simulink model "三相配电系统仿真模型"  (R2024b)
settings: Solver=VariableStepAuto  StartTime=0.0  StopTime=0.5  RelTol=1e-3
libraries: spsCurrentMeasurementLib x18, spsVoltageMeasurementLib x18, spsGroundLib x6, spsThreePhaseSeriesRLCBranchLib x2, spsThreePhaseTransformerThreeWindingsLib x2, spsThreePhaseSeriesRLCLoadLib x1, spsThreePhaseSourceLib x1, sps_lib x1
settings Model: Creator=Land  LastModifiedBy=MihoLocal
settings SFSimCC: UsePrecompiledLibraries=Avoid  SimTargetLang=C++  GPUAcceleration=on  SimDLTargetLibrary=cudnn

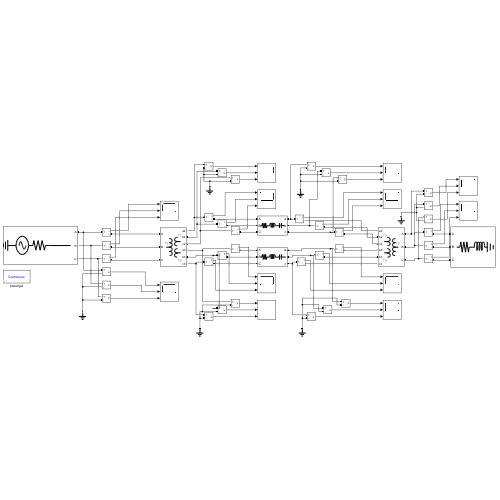
[thumbnail: Simulink's stored preview of the top-level diagram]
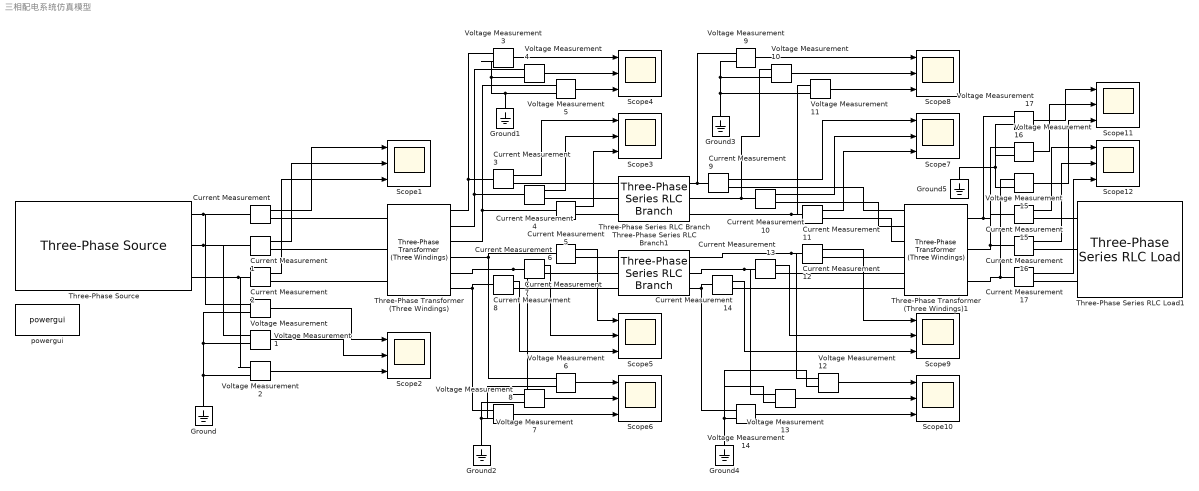
== system 三相配电系统仿真模型 ==
  Current Measurement{,1..17} (18 alike) : spsCurrentMeasurementLib/Current Measurement  PhasorSimulation=off  OutputType=Complex  PSBequivalent=0
  Ground{,1..5} (6 alike) : spsGroundLib/Ground  LConnTagsString=a
  Scope{1..12} (12 alike) : Scope  NumInputPorts=3
  Three-Phase Series RLC Branch : spsThreePhaseSeriesRLCBranchLib/Three-Phase Series RLC Branch  LConnTagsString=A|B|C  RConnTagsString=A|B|C  BranchType=RLC  Resistance=5  Inductance=1e-3  Capacitance=0  Measurements=None
  Three-Phase Series RLC Branch1 : spsThreePhaseSeriesRLCBranchLib/Three-Phase Series RLC Branch  LConnTagsString=A|B|C  RConnTagsString=A|B|C  BranchType=RLC  Resistance=5  Inductance=1e-3  Capacitance=1e-3  Measurements=None
  Three-Phase Series RLC Load1 : spsThreePhaseSeriesRLCLoadLib/Three-Phase Series RLC Load  LConnTagsString=A|B|C  Configuration=Y (grounded)  NominalVoltage=30  Vabc=[1e3 1e3 1e3]  Vabcp=[1e3 1e3 1e3]  NominalFrequency=50  UnbalancedPower=off  ActivePower=10e3  InductivePower=1  CapacitivePower=0  Pabc=[10e3 9e3 11e3]  QLabc=[100 90 110]  QCabc=[100 90 110]  Pabcp=[10e3 9e3 11e3]  QLabcp=[100 90 110]  QCabcp=[100 90 110]  Measurements=None  LoadType=constant Z
  Three-Phase Transformer (Three Windings) : spsThreePhaseTransformerThreeWindingsLib/Three-Phase Transformer (Three Windings)  Winding1Connection=Yg  Winding2Connection=Yg  Winding3Connection=Yg  CoreType=Three single-phase transformers  SetSaturation=off  Hysteresis=off  DataFile='hysteresis'  SetInitialFlux=off  Measurements=None  UNITS=pu  NominalPower=[ 24 , 50 ]  Winding1=[ 12 , 0.002 , 0.08 ]  Winding2=[ 12 , 0.002 , 0.08 ]  Winding3=[ 12 , 0.002 , 0.08 ]  Rm=500  Lm=500  L0=0.5  Saturation=[ 0,0 ; 0.0024,1.2 ; 1.0,1.52 ]  InitialFluxes=[0.8 -0.8 0.7]  BreakLoop=off  DiscreteSolver=Trapezoidal iterative  DataType=off  TransfoNumber=1
      settings: LibrarySourceBlock=|
      | sps_lib/Power Grid Elements/Three-Phase
      | Transformer
      | (Three Windings)
  Three-Phase Transformer (Three Windings)1 : spsThreePhaseTransformerThreeWindingsLib/Three-Phase Transformer (Three Windings)  Winding1Connection=Yg  Winding2Connection=Yg  Winding3Connection=Yg  CoreType=Three single-phase transformers  SetSaturation=off  Hysteresis=off  DataFile='hysteresis'  SetInitialFlux=off  Measurements=None  UNITS=pu  NominalPower=[ 24 , 50 ]  Winding1=[ 12 , 0.002 , 0.08 ]  Winding2=[ 12 , 0.002 , 0.08 ]  Winding3=[ 12 , 0.002 , 0.08 ]  Rm=500  Lm=500  L0=0.5  Saturation=[ 0,0 ; 0.0024,1.2 ; 1.0,1.52 ]  InitialFluxes=[0.8 -0.8 0.7]  BreakLoop=off  DiscreteSolver=Trapezoidal iterative  DataType=off  TransfoNumber=1
      settings: LibrarySourceBlock=|
      | sps_lib/Power Grid Elements/Three-Phase
      | Transformer
      | (Three Windings)
  Three-Phase Source : spsThreePhaseSourceLib/Three-Phase Source  InternalConnection=Yg  VoltagePhases=off  Voltage=12  PhaseAngle=0  Voltage_phases=[25e3 25e3 25e3]/sqrt(3)  PhaseAngles_phases=[0 -120 +120]  Frequency=50  NonIdealSource=on  SpecifyImpedance=off  Resistance=1  Inductance=0  ShortCircuitLevel=100e6  BaseVoltage=0  XRratio=7  BusType=swing  Pref=10e3  Qref=0  Prefabc=[10e3, 10e3, 10e3]  Qrefabc=[0, 0, 0]  Qmin=-inf  Qmax=inf
  Voltage Measurement{,1..17} (18 alike) : spsVoltageMeasurementLib/Voltage Measurement  PhasorSimulation=off  OutputType=Complex  PSBequivalent=0
  powergui : sps_lib/powergui  Priority=1  SimulationMode=Continuous  SampleTime=50e-6  frequency=60  Iterations=50  frequencyindice=50  Pbase=100e6  ErrMax=1e-4  UnitsV=kV  UnitsW=MW  buscounter=0  FunctionMessages=off  echomessages=off  EnableUseOfTLC=off  CurrentSourceSwitches=off  DisableSnubberDevices=off  DisableRonSwitches=off  DisableVfSwitches=off  DisplayEquations=off  AutomaticDiscreteSolvers=off  SolverType=Tustin/Backward Euler (TBE)  Interpol=off  ExternalGateDelay=off  methode=off  Ts=100  x0status=blocks  SPID=on  SwTol=0  HookPort=off  NonlinearTolerance=1e-4  nMaxIteration=100  ContinueOnMaxIteration=off  RestoreLinks=warning  ResistiveCurrentMeasurement=off  Frange=[0:2:500]  Ylog=off  Xlog=on  ShowGrid=off  save=off  variable=ZData  structure=0  ZoomFFT=off  StartTime=0.0  cycles=1  DisplayStyle=1  fundamental=60  FreqAxis=off  MaxFrequency=1000  frequencyindicesteady=1  RmsSteady=1  display=off
  wires:
  Current Measurement/1 -> Scope1/1
  Current Measurement1/1 -> Scope1/2
  Current Measurement2/1 -> Scope1/3
  Voltage Measurement/1 -> Scope2/1
  Voltage Measurement1/1 -> Scope2/2
  Voltage Measurement2/1 -> Scope2/3
  Current Measurement3/1 -> Scope3/1
  Current Measurement4/1 -> Scope3/2
  Current Measurement5/1 -> Scope3/3
  Voltage Measurement3/1 -> Scope4/1
  Voltage Measurement4/1 -> Scope4/2
  Voltage Measurement5/1 -> Scope4/3
  Current Measurement6/1 -> Scope5/1
  Current Measurement7/1 -> Scope5/2
  Current Measurement8/1 -> Scope5/3
  Voltage Measurement6/1 -> Scope6/1
  Voltage Measurement7/1 -> Scope6/2
  Voltage Measurement8/1 -> Scope6/3
  Voltage Measurement9/1 -> Scope8/1
  Voltage Measurement10/1 -> Scope8/2
  Voltage Measurement11/1 -> Scope8/3
  Current Measurement9/1 -> Scope7/1
  Current Measurement10/1 -> Scope7/2
  Current Measurement11/1 -> Scope7/3
  Current Measurement12/1 -> Scope9/1
  Current Measurement13/1 -> Scope9/2
  Current Measurement14/1 -> Scope9/3
  Voltage Measurement13/1 -> Scope10/2
  Voltage Measurement14/1 -> Scope10/3
  Voltage Measurement12/1 -> Scope10/1
  Voltage Measurement17/1 -> Scope11/1
  Voltage Measurement16/1 -> Scope11/2
  Voltage Measurement15/1 -> Scope11/3
  Current Measurement15/1 -> Scope12/1
  Current Measurement16/1 -> Scope12/2
  Current Measurement17/1 -> Scope12/3
  connections:
  Three-Phase Source/RConn2 -- Current Measurement1/LConn1 -- Voltage Measurement1/LConn1
  Current Measurement2/LConn1 -- Three-Phase Source/RConn3 -- Voltage Measurement2/LConn1
  Three-Phase Source/RConn1 -- Voltage Measurement/LConn1 -- Current Measurement/LConn1
  Current Measurement/RConn1 -- Three-Phase Transformer (Three Windings)/LConn1
  Current Measurement1/RConn1 -- Three-Phase Transformer (Three Windings)/LConn2
  Current Measurement2/RConn1 -- Three-Phase Transformer (Three Windings)/LConn3
  Voltage Measurement1/LConn2 -- Voltage Measurement/LConn2 -- Ground/LConn1 -- Voltage Measurement2/LConn2
  Current Measurement3/RConn1 -- Three-Phase Series RLC Branch/LConn1
  Current Measurement4/RConn1 -- Three-Phase Series RLC Branch/LConn2
  Current Measurement5/RConn1 -- Three-Phase Series RLC Branch/LConn3
  Three-Phase Transformer (Three Windings)/RConn1 -- Voltage Measurement3/LConn1 -- Current Measurement3/LConn1
  Current Measurement4/LConn1 -- Voltage Measurement4/LConn1 -- Three-Phase Transformer (Three Windings)/RConn2
  Three-Phase Transformer (Three Windings)/RConn3 -- Voltage Measurement5/LConn1 -- Current Measurement5/LConn1
  Voltage Measurement3/LConn2 -- Voltage Measurement4/LConn2 -- Ground1/LConn1 -- Voltage Measurement5/LConn2
  Current Measurement8/RConn1 -- Three-Phase Series RLC Branch1/LConn3
  Current Measurement7/RConn1 -- Three-Phase Series RLC Branch1/LConn2
  Current Measurement6/RConn1 -- Three-Phase Series RLC Branch1/LConn1
  Three-Phase Transformer (Three Windings)/RConn4 -- Voltage Measurement6/LConn1 -- Current Measurement6/LConn1
  Three-Phase Transformer (Three Windings)/RConn5 -- Voltage Measurement7/LConn1 -- Current Measurement7/LConn1
  Current Measurement8/LConn1 -- Voltage Measurement8/LConn1 -- Three-Phase Transformer (Three Windings)/RConn6
  Voltage Measurement8/LConn2 -- Voltage Measurement6/LConn2 -- Voltage Measurement7/LConn2 -- Ground2/LConn1
  Current Measurement9/LConn1 -- Voltage Measurement9/LConn1 -- Three-Phase Series RLC Branch/RConn1
  Three-Phase Series RLC Branch/RConn2 -- Voltage Measurement10/LConn1 -- Current Measurement10/LConn1
  Three-Phase Series RLC Branch/RConn3 -- Voltage Measurement11/LConn1 -- Current Measurement11/LConn1
  Current Measurement9/RConn1 -- Three-Phase Transformer (Three Windings)1/RConn1
  Current Measurement10/RConn1 -- Three-Phase Transformer (Three Windings)1/RConn2
  Three-Phase Transformer (Three Windings)1/RConn3 -- Current Measurement11/RConn1
  Voltage Measurement9/LConn2 -- Voltage Measurement10/LConn2 -- Voltage Measurement11/LConn2 -- Ground3/LConn1
  Current Measurement12/RConn1 -- Three-Phase Transformer (Three Windings)1/RConn4
  Current Measurement13/RConn1 -- Three-Phase Transformer (Three Windings)1/RConn5
  Three-Phase Transformer (Three Windings)1/RConn6 -- Current Measurement14/RConn1
  Three-Phase Series RLC Branch1/RConn3 -- Voltage Measurement14/LConn1 -- Current Measurement14/LConn1
  Current Measurement13/LConn1 -- Voltage Measurement13/LConn1 -- Three-Phase Series RLC Branch1/RConn2
  Current Measurement12/LConn1 -- Voltage Measurement12/LConn1 -- Three-Phase Series RLC Branch1/RConn1
  Ground4/LConn1 -- Voltage Measurement12/LConn2 -- Voltage Measurement13/LConn2 -- Voltage Measurement14/LConn2
  Current Measurement15/RConn1 -- Three-Phase Series RLC Load1/LConn1
  Current Measurement15/LConn1 -- Voltage Measurement17/LConn1 -- Three-Phase Transformer (Three Windings)1/LConn1
  Current Measurement16/RConn1 -- Three-Phase Series RLC Load1/LConn2
  Current Measurement16/LConn1 -- Voltage Measurement16/LConn1 -- Three-Phase Transformer (Three Windings)1/LConn2
  Three-Phase Series RLC Load1/LConn3 -- Current Measurement17/RConn1
  Current Measurement17/LConn1 -- Voltage Measurement15/LConn1 -- Three-Phase Transformer (Three Windings)1/LConn3
  Voltage Measurement15/LConn2 -- Voltage Measurement17/LConn2 -- Voltage Measurement16/LConn2 -- Ground5/LConn1
